simulink model "scen3_PD"  (R2022a)
settings: Solver=ode4  StartTime=0.0  StopTime=tsim*1.64  FixedStep=0.01  RelTol=1e-3
undefined symbols (not defined in the file): des_z, Kd, Kp, noise, Q, saturation_on, trajectory
libraries: dspmtrx3 x2, dspindex x1
settings Model: Creator=PC  LastModifiedBy=PC
settings SolverCC: AlgebraicLoopSolver=TrustRegion
settings DataIOCC: ReturnWorkspaceOutputs=off
settings DebuggingCC: UnconnectedInputMsg=warning  UnconnectedOutputMsg=warning  UnconnectedLineMsg=warning  SFMachineParentedDataDiag=warning  UnderSpecifiedDimensionMsg=warning
settings RTWCC: DLArmComputeVersion=19.05

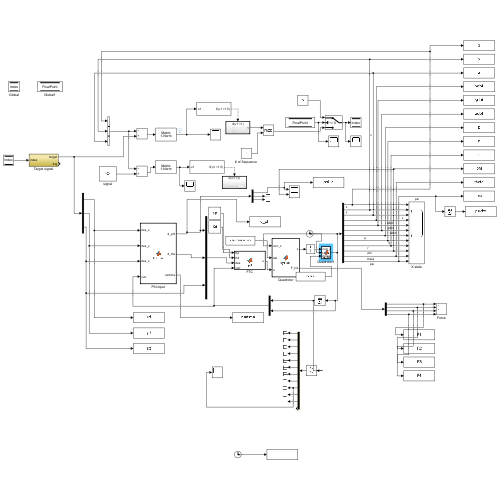
[thumbnail: Simulink's stored preview of the top-level diagram]
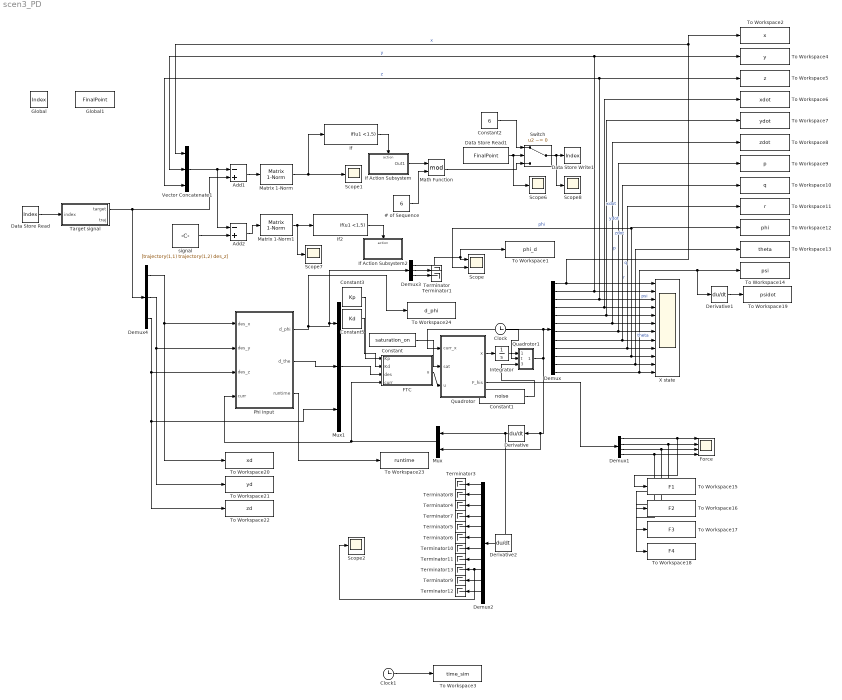
== system scen3_PD ==
  "# of Sequence " : Constant  Value=6
  Add1 : Sum  Inputs=-+
  Add2 : Sum  Inputs=-+
  Clock : Clock
  Clock1 : Clock
  Constant : Constant  Value=saturation_on
  Constant1 : Constant  Value=noise
  Constant2 : Constant  Value=6
  Constant3 : Constant  Value=Kp
  Constant5 : Constant  Value=Kd
  Data Store Read : DataStoreRead  DataStoreName=Index  IndexOptions=Index vector (dialog)  Indices=1  OutputSizes=1
  Data Store Read1 : DataStoreRead  DataStoreName=FinalPoint  IndexOptions=Index vector (dialog)  Indices=1  OutputSizes=1
  Data Store Write1 : DataStoreWrite  DataStoreName=Index  IndexOptions=Index vector (dialog)  Indices=1  OutputSizes=1
  Demux : Demux  Outputs=12
  Demux1 : Demux
  Demux2 : Demux  Outputs=12
  Demux3 : Demux  Outputs=3
  Demux4 : Demux  Outputs=3
  Derivative : Derivative
  Derivative1 : Derivative
  Derivative2 : Derivative
  FTC : MATLAB Function  TreatAsAtomicUnit=on
  Force : Scope  NumInputPorts=4
  Global : DataStoreMemory  DataStoreName=Index  ReadBeforeWriteMsg=warning  WriteAfterWriteMsg=warning  WriteAfterReadMsg=warning  ShowAdditionalParam=off  OutDataTypeStr=double
  Global1 : DataStoreMemory  DataStoreName=FinalPoint  ReadBeforeWriteMsg=warning  WriteAfterWriteMsg=warning  WriteAfterReadMsg=warning  ShowAdditionalParam=off  OutDataTypeStr=double
  If : If  IfExpression=u1 <1.5  ShowElse=off
  If Action Subsystem : Subsystem  TreatAsAtomicUnit=on
  If Action Subsystem2 : Subsystem  TreatAsAtomicUnit=on
  If2 : If  IfExpression=u1 <1.5  ShowElse=off
  Integrator : Integrator  InitialCondition=Q.init
  Math Function : Math  Operator=mod  SignedPower=on
  Matrix 1-Norm : dspmtrx3/Matrix  1-Norm  roundingMode=Floor  overflowMode=off  outputDataTypeStr=Inherit: Same as accumulator  outputMin=[]  outputMax=[]  outputLastDataTypeStr=Inherit: Same as accumulator
      settings: SourceProductBaseCode=DS
  Matrix 1-Norm1 : dspmtrx3/Matrix  1-Norm  roundingMode=Floor  overflowMode=off  outputDataTypeStr=Inherit: Same as accumulator  outputMin=[]  outputMax=[]  outputLastDataTypeStr=Inherit: Same as accumulator
      settings: SourceProductBaseCode=DS
  Mux : Mux  Inputs=2
  Mux1 : Mux  Inputs=3
  Phi input : MATLAB Function  TreatAsAtomicUnit=on
  Quadrotor : MATLAB Function  TreatAsAtomicUnit=on
  Quadrotor1 : MATLAB Function  TreatAsAtomicUnit=on
  Scope : Scope  NumInputPorts=2
  Scope{1..2,6..8} (5 alike) : Scope
  Switch : Switch  Criteria=u2 ~= 0  SaturateOnIntegerOverflow=off  InputSameDT=off
  Target signal : Subsystem
  Terminator{,1,3..13} (13 alike) : Terminator
  To Workspace1 : ToWorkspace  VariableName=phi_d  SampleTime=-1
      settings: Save2DSignal=2-D array (concatenate along first dimension)
  To Workspace10 : ToWorkspace  VariableName=q  SampleTime=-1
      settings: Save2DSignal=2-D array (concatenate along first dimension)
  To Workspace11 : ToWorkspace  VariableName=r  SampleTime=-1
      settings: Save2DSignal=2-D array (concatenate along first dimension)
  To Workspace12 : ToWorkspace  VariableName=phi  SampleTime=-1
      settings: Save2DSignal=2-D array (concatenate along first dimension)
  To Workspace13 : ToWorkspace  VariableName=theta  SampleTime=-1
      settings: Save2DSignal=2-D array (concatenate along first dimension)
  To Workspace14 : ToWorkspace  VariableName=psi  SampleTime=-1
      settings: Save2DSignal=2-D array (concatenate along first dimension)
  To Workspace15 : ToWorkspace  VariableName=F1  SampleTime=-1
      settings: Save2DSignal=2-D array (concatenate along first dimension)
  To Workspace16 : ToWorkspace  VariableName=F2  SampleTime=-1
      settings: Save2DSignal=2-D array (concatenate along first dimension)
  To Workspace17 : ToWorkspace  VariableName=F3  SampleTime=-1
      settings: Save2DSignal=2-D array (concatenate along first dimension)
  To Workspace18 : ToWorkspace  VariableName=F4  SampleTime=-1
      settings: Save2DSignal=2-D array (concatenate along first dimension)
  To Workspace19 : ToWorkspace  VariableName=psidot  SampleTime=-1
      settings: Save2DSignal=2-D array (concatenate along first dimension)
  To Workspace2 : ToWorkspace  VariableName=x  SampleTime=-1
      settings: Save2DSignal=2-D array (concatenate along first dimension)
  To Workspace20 : ToWorkspace  VariableName=xd  SampleTime=-1
      settings: Save2DSignal=2-D array (concatenate along first dimension)
  To Workspace21 : ToWorkspace  VariableName=yd  SampleTime=-1
      settings: Save2DSignal=2-D array (concatenate along first dimension)
  To Workspace22 : ToWorkspace  VariableName=zd  SampleTime=-1
      settings: Save2DSignal=2-D array (concatenate along first dimension)
  To Workspace23 : ToWorkspace  VariableName=runtime  SampleTime=-1
      settings: Save2DSignal=2-D array (concatenate along first dimension)
  To Workspace24 : ToWorkspace  VariableName=d_phi  SampleTime=-1
      settings: Save2DSignal=2-D array (concatenate along first dimension)
  To Workspace3 : ToWorkspace  VariableName=time_sim  SampleTime=-1
      settings: Save2DSignal=2-D array (concatenate along first dimension)
  To Workspace4 : ToWorkspace  VariableName=y  SampleTime=-1
      settings: Save2DSignal=2-D array (concatenate along first dimension)
  To Workspace5 : ToWorkspace  VariableName=z  SampleTime=-1
      settings: Save2DSignal=2-D array (concatenate along first dimension)
  To Workspace6 : ToWorkspace  VariableName=xdot  SampleTime=-1
      settings: Save2DSignal=2-D array (concatenate along first dimension)
  To Workspace7 : ToWorkspace  VariableName=ydot  SampleTime=-1
      settings: Save2DSignal=2-D array (concatenate along first dimension)
  To Workspace8 : ToWorkspace  VariableName=zdot  SampleTime=-1
      settings: Save2DSignal=2-D array (concatenate along first dimension)
  To Workspace9 : ToWorkspace  VariableName=p  SampleTime=-1
      settings: Save2DSignal=2-D array (concatenate along first dimension)
  Vector Concatenate1 : Concatenate  NumInputs=3
  X state : Scope  NumInputPorts=12
  signal : Constant  Value=[trajectory(1,1) trajectory(1,2) des_z]  VectorParams1D=off
  wires:
  Mux1/1 -> FTC/3(des)
  Demux/3 -> X state/3, To Workspace5/1, Vector Concatenate1/3  "z"
  Demux/4 -> X state/4, To Workspace6/1  "xdot"
  Demux/5 -> X state/5, To Workspace7/1  "ydot"
  Demux/6 -> X state/6, To Workspace8/1  "zdot"
  Demux/7 -> X state/7, To Workspace9/1  "p"
  Demux/8 -> X state/8, To Workspace10/1  "q"
  Demux/9 -> X state/9, To Workspace11/1  "r"
  Demux/10 -> X state/10, To Workspace12/1, Scope/2  "phi"
  Demux/11 -> X state/11, To Workspace13/1  "theta"
  FTC/1(u) -> Quadrotor/3(u)
  Mux/1 -> FTC/4(curr), Phi input/4(curr)
  Derivative/1 -> Mux/1, Derivative2/1
  Derivative2/1 -> Demux2/1
  Phi input/2(d_the) -> Mux1/2
  Demux2/1 -> Terminator3/1
  Demux2/2 -> Terminator8/1
  Demux2/3 -> Terminator4/1
  Demux2/4 -> Terminator7/1
  Demux2/5 -> Terminator5/1
  Demux2/6 -> Terminator6/1
  Demux2/10 -> Terminator9/1
  Demux2/7 -> Terminator10/1
  Demux2/8 -> Terminator11/1
  Demux2/11 -> Terminator12/1
  Demux2/9 -> Scope2/1, Terminator13/1
  Demux4/3 -> To Workspace22/1, Mux1/3, Phi input/3(des_z)
  Quadrotor/2(F_his) -> Demux1/1
  Demux1/1 -> To Workspace15/1, Force/1
  Demux1/3 -> To Workspace17/1, Force/3
  Demux1/4 -> To Workspace18/1, Force/4
  Demux1/2 -> Force/2, To Workspace16/1
  Clock1/1 -> To Workspace3/1
  Demux/12 -> X state/12, Derivative1/1, To Workspace14/1  "psi"
  Derivative1/1 -> To Workspace19/1
  Phi input/1(d_phi) -> To Workspace24/1, Demux3/1, Mux1/1
  Demux3/1 -> To Workspace1/1, Scope/1
  Constant/1 -> Quadrotor/2(sat)
  Data Store Read/1 -> Target signal/1(index)
  "# of Sequence "/1 -> Math Function/2
  Target signal/1(target) -> Demux4/1, Add1/2
  If Action Subsystem/1(Out1) -> Math Function/1
  Add1/1 -> Matrix 1-Norm/1
  Demux4/1 -> To Workspace20/1, Phi input/1(des_x)
  Demux4/2 -> To Workspace21/1, Phi input/2(des_y)
  Vector Concatenate1/1 -> Add2/1, Add1/1
  signal/1 -> Add2/2
  Matrix 1-Norm1/1 -> If2/1, Scope7/1
  Add2/1 -> Matrix 1-Norm1/1
  If2/1 -> If Action Subsystem2/Action
  Data Store Read1/1 -> Scope6/1, Switch/2
  Switch/1 -> Scope8/1, Data Store Write1/1
  Math Function/1 -> Switch/3
  Constant2/1 -> Switch/1
  Constant3/1 -> FTC/1(Kp)
  If/1 -> If Action Subsystem/Action
  Demux3/2 -> Terminator/1
  Demux3/3 -> Terminator1/1
  Phi input/3(runtime) -> To Workspace23/1
  Demux/2 -> X state/2, To Workspace4/1, Vector Concatenate1/2  "y"
  Demux/1 -> X state/1, Vector Concatenate1/1, To Workspace2/1  "x"
  Matrix 1-Norm/1 -> Scope1/1, If/1
  Quadrotor/1(x) -> Integrator/1
  Integrator/1 -> Quadrotor1/1(curr_x)
  Quadrotor1/1(x) -> Quadrotor/1(curr_x), Demux/1, Mux/2, Derivative/1
  Constant1/1 -> Quadrotor1/3(noise)
  Clock/1 -> Quadrotor1/2(t)
  Constant5/1 -> FTC/2(Kd)

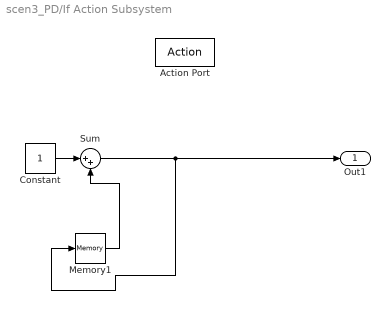
== system scen3_PD/If Action Subsystem ==
  Action Port : ActionPort  ActionPortLabel=if(u1 <1.5)
  Constant : Constant
  Memory1 : Memory
  Sum : Sum  Inputs=|++
  Out1 : Outport  VectorParamsAs1DForOutWhenUnconnected=off
  wires:
  Memory1/1 -> Sum/2
  Constant/1 -> Sum/1
  Sum/1 -> Memory1/1, Out1/1

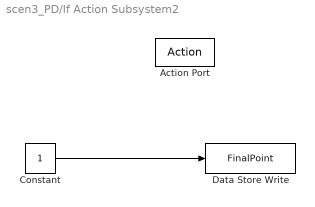
== system scen3_PD/If Action Subsystem2 ==
  Action Port : ActionPort  ActionPortLabel=if(u1 <1.5)
  Constant : Constant
  Data Store Write : DataStoreWrite  DataStoreName=FinalPoint  IndexOptions=Index vector (dialog)  Indices=1  OutputSizes=1
  wires:
  Constant/1 -> Data Store Write/1

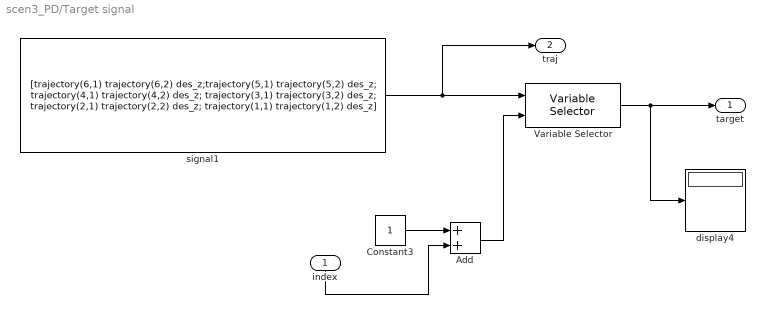
== system scen3_PD/Target signal ==
  index : Inport
  Add : Sum
  Constant3 : Constant
  Variable Selector : dspindex/Variable Selector  NumInputs=1  rowsOrCols=Rows  IdxMode=Variable  Elements=[1 3]  ZerOneIdxMode=One-based  errmode=Clip Index  FillMode=on  FillValues=0
  display4 : Display
  signal1 : Constant  Value=[trajectory(6,1) trajectory(6,2) des_z;trajectory(5,1) trajectory(5,2) des_z; trajectory(4,1) trajectory(4,2) des_z; trajectory(3,1) trajectory(3,2) des_z; trajectory(2,1) trajectory(2,2) des_z; trajectory(1,1) trajectory(1,2) des_z]  VectorParams1D=off
  target : Outport  VectorParamsAs1DForOutWhenUnconnected=off
  traj : Outport  Port=2  VectorParamsAs1DForOutWhenUnconnected=off
  wires:
  Add/1 -> Variable Selector/2
  Variable Selector/1 -> target/1, display4/1
  index/1 -> Add/2
  signal1/1 -> traj/1, Variable Selector/1
  Constant3/1 -> Add/1

== matlab function scen3_PD/Quadrotor1 ==
  settings: updateMethod=DISCRETE
  data: curr_x input; t input; x output; noise input
function x  = system(curr_x, t, noise)

ind = fix(t/0.01)+1;
% mu = 0;
% sigma = 0.054;



x = curr_x;
x(1) = curr_x(1)+noise(ind,1);
x(2) = curr_x(2)+noise(ind,2);
x(3) = curr_x(3)+noise(ind,3);

== matlab function scen3_PD/Quadrotor ==
  settings: updateMethod=DISCRETE
  data: curr_x input; sat input; u input; x output; F_his output
function [x,F_his] = system(curr_x,sat,u)
% x = {xyz xyzvel pqr phi theta psi}
x = zeros(12,1);
% Properties
m = 1.282; g = 9.81;
Ix = 4.856*10^-3; Iy = Ix; Iz = 8.801*10^-3;
b = 0.0066;
kr = 0.02;
kt = 0.5;
l = 0.1;

u_temp = zeros(3,1);
u_temp = u;
u = u_temp;

T = u(1); tp = u(2); tq = u(3);% tr = u(4);
tr = b*(T-2*tp/l);
A = [1 1 1; 0 l 0;-l 0 l];

F=inv(A)*[T tp tq]';

f1 = F(1); f2 = F(2); f3 = F(3);
ub = m*g;
lb = 0;

saturation1_lb = 0;
saturation1_ub = 0;
saturation2_lb = 0;
saturation2_ub = 0;
saturation3_lb = 0;
saturation3_ub = 0;
saturation1_lb_margin = 0;
saturation1_ub_margin = 0;
saturation2_lb_margin = 0;
saturation2_ub_margin = 0;
saturation3_lb_margin = 0;
saturation3_ub_margin = 0;

sat = 0; 
if sat == 1
    if f1 < lb
        saturation1_lb = abs(lb - f1);
        saturation1_lb_margin = abs(lb - f1);
        f1 = lb;
    else
        saturation1_lb_margin = lb - f1;
    end
    
    if f1 > ub
        saturation1_ub = abs(ub - f1);
        saturation1_ub_margin = abs(ub - f1);
        f1 = ub;
    else
        saturation1_ub_margin = f1 - ub;
    end
    
    if f2 < lb
        saturation2_lb = abs(lb - f2);
        saturation2_lb_margin = abs(lb - f2);
        f2 = lb;
    else
        saturation2_lb_margin = lb - f2;
    end
    
    if f2 > ub
        saturation2_ub = abs(ub - f2);
        saturation2_ub_margin = abs(ub - f2);
        f2 = ub;
    else
        saturation2_ub_margin = f2 - ub;
    end
    
    if f3 < lb
        saturation3_lb = abs(lb - f3);
        saturation3_lb_margin = abs(lb - f3);
        f3 = lb;
    else
        saturation3_lb_margin = lb - f3;
    end
    
    if f3 > ub
        saturation3_ub = abs(ub - f3);
        saturation3_ub_margin = abs(ub - f3);
        f3 = ub;
    else
        saturation3_ub_margin = f3 - ub;
    end
end

saturation = max([saturation1_lb,saturation1_ub,saturation2_lb,saturation2_ub,saturation3_lb,saturation3_ub]);
saturation_margin = max([saturation1_lb_margin,saturation1_ub_margin,saturation2_lb_margin,saturation2_ub_margin,saturation3_lb_margin,saturation3_ub_margin]);

f4 = 0;
F_his = [f1 f2 f3 f4]';
T = f1+f2+f3;
tp = l*(f2);
tq = l*(f3-f1);
tr = b*(f1+f3-f2);

% Current state
x1  = curr_x(1);
x2  = curr_x(2);
x3  = curr_x(3);
x4  = curr_x(4);
x5  = curr_x(5);
x6  = curr_x(6);
x7  = curr_x(7);
x8  = curr_x(8);
x9  = curr_x(9);
x10 = curr_x(10);
x11 = curr_x(11);
x12 = curr_x(12);

% Position
x(1) = x4;
x(2) = x5;
x(3) = x6;


% Velocity
x(4) = T/m*(cos(x12)*sin(x11)*cos(x10) + sin(x12)*sin(x10)) - kt/m*x4;
x(5) = T/m*(sin(x12)*sin(x11)*cos(x10) - cos(x12)*sin(x10)) - kt/m*x5;
x(6) = -g + T*(1/m)*(cos(x10)*cos(x11)) - kt/m*x6;
% Body rate
x(7) = ((Ix-Iz)*x8*x9 + tp)/Ix;
x(8) = ((Iz-Ix)*x7*x9 + tq)/Ix;
x(9) = (-kr*x9 + tr)/Iz;
% Angle
x(10) = x7 + x8*sin(x10)*tan(x11) + x9*cos(x10)*tan(x11);
x(11) = x8*cos(x10) - x9*sin(x10);
x(12) = x8*sin(x10)/cos(x11) + x9*cos(x10)*cos(x11);

if x3<=0
    B=1;
else
    B=0;
end

== matlab function scen3_PD/Phi input ==
  settings: updateMethod=DISCRETE
  data: des_x input; des_y input; des_z input; d_phi output; d_the output; curr input; runtime output
function [d_phi,d_the,runtime]  = fcn_ref( des_x,des_y,des_z,curr)
    tic;
    m = 1.282; g = 9.81;
    Ix = 4.856*10^-3; Iy = Ix; Iz = 8.801*10^-3;
    b = 0.0066;
    kr = 0.02; %drag coefficient
    kt = 0.5;
    l = 0.1;
    
    delta_t = 0.01;
    
    % current state_dot
    N = 0;
    xdot   = curr(N+1); ydot   = curr(N+2); zdot   = curr(N+3);
    x2dot  = curr(N+4); y2dot  = curr(N+5); z2dot  = curr(N+6);
    pdot   = curr(N+7); qdot   = curr(N+8); rdot   = curr(N+9);
    phidot = curr(N+10);thedot = curr(N+11);psidot = curr(N+12);
    state_dot = [xdot, ydot, zdot, x2dot, y2dot, z2dot, pdot, qdot, rdot, phidot, thedot, psidot];
    
    % current state
    N = 12;
    x    = curr(N+1); y    = curr(N+2); z    = curr(N+3);
    xdot = curr(N+4); ydot = curr(N+5); zdot = curr(N+6);
    p    = curr(N+7); q    = curr(N+8); r    = curr(N+9);
    phi  = curr(N+10);the  = curr(N+11);psi  = curr(N+12);
    
    while psi > pi
        psi = psi - 2*pi;
    end
    
    while psi < -pi
        psi = psi + 2*pi;
    end
    state = [x, y, z, xdot, ydot, zdot, p, q, r, phi, the, psi];
    
%     des_x = (x+des_x)/2;
%     des_y = (y+des_y)/2;

    % Thrust constraint
    % F_ = F(1)+F(2)+F(3);
    f_max = m*g;
    uf_max = 2*f_max;
    uf_min = f_max;
    up_max = l*(f_max);
    up_min = 0;
    ur_max = b*(uf_max-2/l*up_min);
    ur_min = b*(uf_min-2/l*up_max);

    %%%%%%%%%%%%%%%%%%%%%%%%%%%%%%%
    % Objective function for immediate adjustment
    objective = @(u) computePositionError(state, u, des_x, des_y, des_z, m, g, kt, delta_t, uf_max);
    
    % Initial guess for roll angle (phi)
    u_initial = [0];
    
    % Constraints
    A = [];
    b = [];
    Aeq = [];
    beq = [];
    lb = [0];
    ub = [deg2rad(40)]; %, deg2rad(40)];
    
    % Optimization options
    options = optimoptions('fmincon', 'Display', 'iter', 'Algorithm', 'sqp');
    
    % Solve the optimization problem
    [phi_opt, fval] = fmincon(objective, u_initial, A, b, Aeq, beq, lb, ub, [], options);
     
    % Display the results
    fprintf('Optimal roll angle (phi): %.2f rad\n', phi_opt);

    
    %%%%%%%%%%%%%%%%%%
    objective = @(u) cost(state, u, phi_opt);
    
    % Initial guess for roll angle (phi)
    u_initial = [uf_max, up_max, phi_opt];
    
    % Constraints
    A = [];
    b = [];
    Aeq = [];
    beq = [];
    lb = [uf_min, up_min, -deg2rad(40)];
    ub = [uf_max, up_max, deg2rad(40)];
    nonlcon_fn = @(u) nonlcon(u, state, delta_t);

    % Optimization options
    options = optimoptions('fmincon', 'Display', 'iter', 'Algorithm', 'sqp');
    
    % Solve the optimization problem
    [u_opt, fval] = fmincon(objective, u_initial, A, b, Aeq, beq, lb, ub, nonlcon_fn, options);
     
    % Display the results
    fprintf('Optimal roll angle (phi): %.2f rad\n', u_opt(3));    
%     fprintf('Optimal roll angle (the): %.2f rad\n', u_opt(4));      


    %%%%%%%%%%%%%%%%%%%

    % Define the cost function: min (error in position)
%     error = [des_x - x; des_y - y; des_z - z];    
%     cost_function = @(u) cost(u, state, error, m, g, kt, delta_t, Ix, Iz, kr);
%     
%     phi_max = deg2rad(40); % Maximum roll angle
%     phi_min = -deg2rad(40); % Minimum roll angle
%     lb = [phi_min; uf_min];
%     ub = [phi_max; uf_max];
%     u0 = [0; (uf_min + uf_max) / 2];
%     options = optimoptions('fmincon', 'Algorithm', 'sqp', 'Display', 'off');
%     u_opt = fmincon(cost_function, u0, [], [], [], [], lb, ub, [], options);


  
    phi_d = u_opt(3);
    theta_d = 0; %u_opt(4);
    thedot_d = 0;
    the2dot_d = 0;
    phidot_d = 0;
    phi2dot_d = 0;
    
    d_phi = [phi_d, phidot_d, phi2dot_d]';
    d_the = [theta_d, thedot_d, the2dot_d]';
    
    fprintf('Optimal roll angle (phi): %.2f rad\n', phi_d);
    
    runtime = toc;

end    


% Objective function to compute the position error
function error = cost(x, u, phi_target)
    
    m = 1.282; g = 9.81;
    Ix = 4.856*10^-3; Iy = Ix; Iz = 8.801*10^-3;
    b = 0.0066;
    kr = 0.02; %drag coefficient
    kt = 0.5;
    l = 0.1;
    
    % Compute the position error
    error = 100*(u(3)-phi_target)^2;
    fprintf('error: %.2f \n', error);
end

function [c, ceq] = nonlcon(u, x, delta_t)
    % Constants
    m = 1.282; g = 9.81;
    Ix = 4.856*10^-3; Iy = Ix; Iz = 8.801*10^-3;
    b = 0.0066;
    kr = 0.02; %drag coefficient
    kt = 0.5;
    l = 0.1;
    tr = b*(u(1)-2/l*u(2));
    
    % State Variables
    p = x(7) + (((Ix-Iz)*x(8)*x(9) + u(2))/Ix)*delta_t;
    q = x(8) + (((Iz-Ix)*x(7)*x(9))/Ix)*delta_t;
    r = x(9) + ((-kr * x(9) + tr) / Iz) * delta_t;

    % Nonlinear constraint: u(4) = x(10) + (p + q * sin(x(10)) * tan(x(11)) + r * cos(x(10)) * tan(x(11))) * delta_t
    u3_constraint = x(10) + (p + q * sin(x(10)) * tan(x(11)) + r * cos(x(10)) * tan(x(11))) * delta_t;
    u4_constraint = x(11) + (p*cos(x(10)) - r*sin(x(10))) * delta_t;

    % No inequality constraints
    c = [];

    % Equality constraint
    ceq = [u(3) - u3_constraint]; %, u(4) - u4_constraint];
end


    % Objective function to compute the position error
function error = computePositionError(x, u, x_target, y_target, z_target, m, g, kt, delta_t, T)
    

    T = m*g;
    phi = u(1);
    theta = 0.0;
    
    psi_dot = x(8)*sin(x(10))/cos(x(11)) + x(9)*cos(x(10))*cos(x(11));    % Yaw angle
    psi =  x(12); %+psi_dot*delta_t;


    % Update the velocities based on the dynamics
    x_vel_new = x(4) + (T/m*(cos(psi)*sin(phi)*cos(theta) + sin(psi)*sin(theta)) - kt*x(4))*delta_t;
    y_vel_new = x(5) + (T/m*(sin(psi)*sin(phi)*cos(theta) - cos(psi)*sin(theta)) - kt*x(5))*delta_t;
    z_vel_new = x(6) + (-g + T/m*(cos(phi)*cos(theta)) - kt*x(6))*delta_t;

    % Update the positions based on the velocities
    x_pos_new = x(1) + x_vel_new * delta_t;
    y_pos_new = x(2) + y_vel_new * delta_t;
    z_pos_new = x(3) + z_vel_new * delta_t;

    % Compute the position error
    error = ( x_pos_new- x_target)^2 + (y_pos_new-y_target)^2; %+ 0.1*(z_target - z_pos_new)^2 ;
    fprintf('position error: %.2f \n', error);
end

function u = controller(phi_target, z_target, state, state_dot, Kp, Kd)

    m = 1.282; g = 9.81;
    Ix = 4.856*10^-3; Iy = Ix; Iz = 8.801*10^-3;
    b = 0.0066;
    kr = 0.02;
    kt = 0.5;
    l = 0.1;


    % Extract the state variables
    zdot = state_dot(3);
    phi = state(10);
    the = state(11);
    phidot = state_dot(10);
    thedot = state_dot(11);
    z = state(3);
    p = state(7);
    q = state(8);
    r = state(9);
    

    % Dynamics matrices
    F = [p + q*sin(phi)*tan(the) + r*cos(phi)*tan(the)
     q*cos(phi) - r*sin(phi)
     -(Iz - Iy)*q*r/Ix
     -(Ix - Iz)*p*r/Iy
     -kr*r/Iz
     zdot
     -kt*zdot/m - g];
 
    G = [0 0 0
         0 0 0
         0 1/Ix 0
         0 0 1/Iy
         b/Iz -2*b/(l*Iz) 0
         0 0 0
         cos(phi)*cos(the)/m 0 0];
     
    J = [q*cos(phi)*tan(the)-r*sin(phi)*tan(the) q*sin(phi)*sec(the)^2+r*cos(phi)*sec(the)^2 1 sin(phi)*tan(the) cos(phi)*tan(the) 0 0
         -q*sin(phi)-r*cos(phi) 0 0 cos(phi) -sin(phi) 0 0
         0 0 0 0 0 0 1];
    
    ubar = [0 + Kp*(phi_target-phi) + Kd*(0-phidot)
            0 + Kp*(0-the) + Kd*(0-thedot)
            10*(z_target-z) + (0-zdot)];
        
    % Control output
    u = inv(J * G) * (-J * F + ubar);
end

function x_dot = quadrotor_dynamics(x, u)

    m = 1.282; g = 9.81;
    Ix = 4.856*10^-3; Iy = Ix; Iz = 8.801*10^-3;
    b = 0.0066;
    kr = 0.02;
    kt = 0.5;
    l = 0.1;
    

    % Extract states
    x4 = x(4);
    x5 = x(5);
    x6 = x(6);
    x7 = x(7);
    x8 = x(8);
    x9 = x(9);
    phi = x(10);
    theta = x(11);
    psi = x(12);
    
    % Extract inputs
    T = u(1);
    tp = u(2);
    tq = u(3);
    tr = b*(T-2*tp/l);
    
    % Dynamics equations
    x_dot = zeros(1,12);
    % Position
    x_dot(1) = x4;
    x_dot(2) = x5;
    x_dot(3) = x6;
    
    % Velocity
    x_dot(4) = T/m*(cos(psi)*sin(theta)*cos(phi) + sin(psi)*sin(phi)) - kt*x4;
    x_dot(5) = T/m*(sin(psi)*sin(theta)*cos(phi) - cos(psi)*sin(phi)) - kt*x5;
    x_dot(6) = -g + T/m*(cos(phi)*cos(theta)) - kt*x6;
    
    % Body rate
    x_dot(7) = ((Iy-Iz)*x8*x9 + tp)/Ix;
    x_dot(8) = ((Iz-Ix)*x7*x9 + tq)/Iy;
    x_dot(9) = (-kt*x9 + tr)/Iz;
    
    % Angle
    x_dot(10) = x7 + x8*sin(phi)*tan(theta) + x9*cos(phi)*tan(theta);
    x_dot(11) = x8*cos(phi) - x9*sin(phi);
    x_dot(12) = x8*sin(phi)/cos(theta) + x9*cos(phi)/cos(theta);
end

== matlab function scen3_PD/FTC ==
  data: Kp input; Kd input; des input; u output; curr input
function u = pd(Kp,Kd,des,curr)

m = 1.282; g = 9.81;
Ix = 4.856*10^-3; Iy = Ix; Iz = 8.801*10^-3;
b = 0.0066;
kr = 0.02;
kt = 0.5;
l = 0.1;

% current state
N = 0;
xdot   = curr(N+1); ydot   = curr(N+2); zdot   = curr(N+3);
x2dot  = curr(N+4); y2dot  = curr(N+5); z2dot  = curr(N+6);
pdot   = curr(N+7); qdot   = curr(N+8); rdot   = curr(N+9);
phidot = curr(N+10);thedot = curr(N+11);psidot = curr(N+12);

N = 12;
x    = curr(N+1); y    = curr(N+2); z    = curr(N+3);
xdot = curr(N+4); ydot = curr(N+5); zdot = curr(N+6);
p    = curr(N+7); q    = curr(N+8); r    = curr(N+9);
phi  = curr(N+10);the  = curr(N+11);psi  = curr(N+12);
des_temp = zeros(7,1);
des_temp = des;
des = des_temp;
% desired state
phi_d = des(1);
phidot_d = des(2);
phi2dot_d = des(3);
the_d = des(4);
thedot_d = des(5);
the2dot_d = des(6);
z_d   = des(7);

F = [p + q*sin(phi)*tan(the) + r*cos(phi)*tan(the)
     q*cos(phi) - r*sin(phi)
     -(Iz - Iy)*q*r/Ix
     -(Ix - Iz)*p*r/Iy
     -kr*r/Iz
     zdot
     -kt*zdot/m - g];
 
G = [0 0 0
     0 0 0
     0 1/Ix 0
     0 0 1/Iy
     b/Iz -2*b/(l*Iz) 0
     0 0 0
     cos(phi)*cos(the)/m 0 0];
 
J = [q*cos(phi)*tan(the)-r*sin(phi)*tan(the) q*sin(phi)*sec(the)^2+r*cos(phi)*sec(the)^2 1 sin(phi)*tan(the) cos(phi)*tan(the) 0 0
     -q*sin(phi)-r*cos(phi) 0 0 cos(phi) -sin(phi) 0 0
     0 0 0 0 0 0 1];

ubar = [phi2dot_d + Kp*(phi_d-phi) + Kd*(phidot_d-phidot)
        the2dot_d + Kp*(the_d-the) + Kd*(thedot_d-thedot)
        10*(z_d-z) + (0-zdot)];
    
u = inv(J*G)*(-J*F + ubar);
